simulink model "Model23"  (R2020a)
settings: Solver=VariableStepAuto  StartTime=0.0  StopTime=120  RelTol=1e-3
values from neighbouring files (symbols this model uses):
  b = 50.0    [DD23.sldd]
  m = 1000.0    [DD23.sldd]
settings Model: DataDictionary=DD23.sldd  Creator=HP  LastModifiedBy=HP

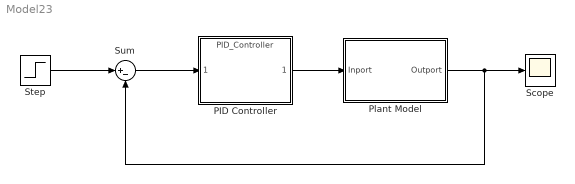
== system Model23 ==
  PID Controller : ModelReference  ModelNameDialog=PID_Controller  ModelReferenceVersion=1.9
  Plant Model : Subsystem
  Scope : Scope
  Step : Step  Time=0  After=u  SampleTime=0
  Sum : Sum  Inputs=|+-
  wires:
  Plant Model/1(Outport) -> Sum/2, Scope/1
  Step/1 -> Sum/1
  Sum/1 -> PID Controller/1
  PID Controller/1 -> Plant Model/1(Inport)

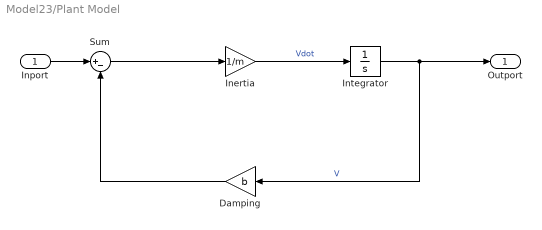
== system Model23/Plant Model ==
  Inport : Inport
  Damping : Gain  Gain=b
  Inertia : Gain  Gain=1/m
  Integrator : Integrator
  Sum : Sum  Inputs=|+-
  Outport : Outport
  wires:
  Sum/1 -> Inertia/1
  Inertia/1 -> Integrator/1  "Vdot"
  Inport/1 -> Sum/1
  Integrator/1 -> Outport/1, Damping/1  "V"
  Damping/1 -> Sum/2
